simulink subsystem "Force_algebraic_estimator"  (R2021a)
settings: Solver=VariableStepAuto  StartTime=0.0  StopTime=10.0  RelTol=1e-3
values from neighbouring files (symbols this model uses):
  Af = 1.6    [kf_dict.sldd]
  Cd = 0.3    [kf_dict.sldd]
  rho_air = 1.206    [kf_dict.sldd]
undefined symbols (not defined in the file or in its folder): g, h, l, lf, lr, M, re
settings Model: Creator=Henrique Mesquita  LastModifiedBy=Henrique Mesquita

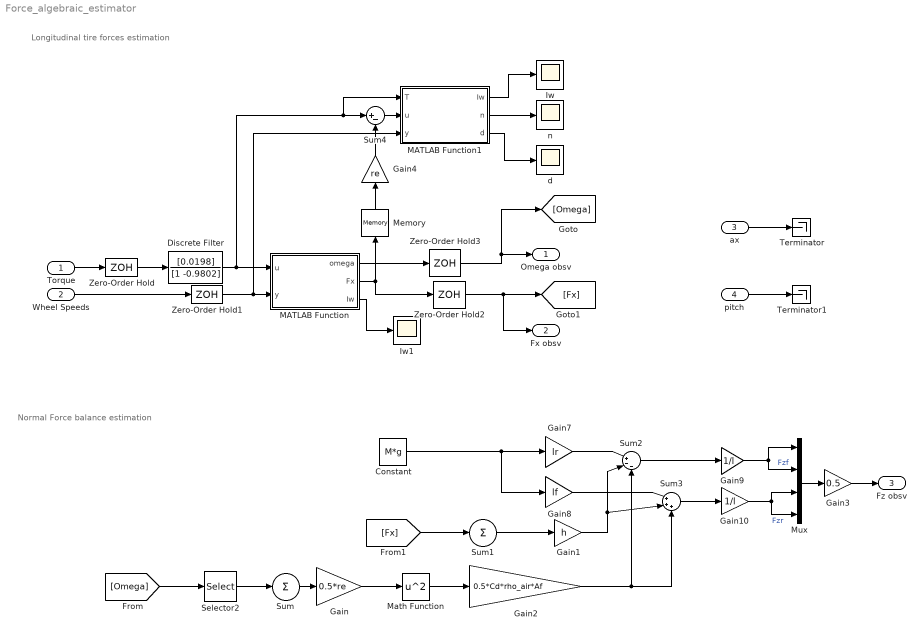
== system Force_algebraic_estimator ==
  note: Longitudinal tire forces estimation
  note: Normal Force balance estimation
  Torque : Inport  PortDimensions=4
  Wheel Speeds : Inport  Port=2  PortDimensions=4
  ax : Inport  Port=3  PortDimensions=1
  pitch : Inport  Port=4  PortDimensions=1
  Constant : Constant  Value=M*g
  Discrete Filter : DiscreteFilter  Numerator=[0.0198]  Denominator=[1 -0.9802]  SampleTime=0.001
  Gain : Gain  Gain=0.5*re
  Gain1 : Gain  Gain=h
  Gain10 : Gain  Gain=1/l
  Gain2 : Gain  Gain=0.5*Cd*rho_air*Af
  Gain3 : Gain  Gain=0.5
  Gain4 : Gain  Gain=re
  Gain7 : Gain  Gain=lr
  Gain8 : Gain  Gain=lf
  Gain9 : Gain  Gain=1/l
  Iw : Scope
  Iw1 : Scope
  MATLAB Function : MATLAB Function  TreatAsAtomicUnit=on
  MATLAB Function1 : MATLAB Function  TreatAsAtomicUnit=on
  Math Function : Math  Operator=square  SaturateOnIntegerOverflow=on
  Memory : Memory  LinearizeAsDelay=on
  Mux : Mux
  Selector2 : Selector  InputPortWidth=4  IndexOptions=Index vector (dialog)  Indices=[1 2]  OutputSizes=1
  Sum : Sum  Inputs=+
  Sum1 : Sum  Inputs=+
  Sum2 : Sum  Inputs=|+--
  Sum3 : Sum  Inputs=|+++
  Sum4 : Sum  Inputs=|+-
  Terminator : Terminator
  Terminator1 : Terminator
  Zero-Order Hold{,1..3} (4 alike) : ZeroOrderHold  SampleTime=0.001
  d : Scope
  n : Scope
  Omega obsv : Outport
  Fx obsv : Outport  Port=2
  Fz obsv : Outport  Port=3
  wires:
  Wheel Speeds/1 -> Zero-Order Hold1/1
  Zero-Order Hold2/1 -> [Fx], Fx obsv/1
  Zero-Order Hold3/1 -> Omega obsv/1, [Omega]
  ax/1 -> Terminator/1
  pitch/1 -> Terminator1/1
  [Omega] -> Selector2/1
  [Fx] -> Sum1/1
  Selector2/1 -> Sum/1
  Sum1/1 -> Gain1/1
  Sum/1 -> Gain/1
  Mux/1 -> Gain3/1
  Sum3/1 -> Gain10/1
  Gain10/1 -> Mux/3, Mux/4  "Fzr"
  Sum2/1 -> Gain9/1
  Gain1/1 -> Sum2/2, Sum3/2
  Gain9/1 -> Mux/1, Mux/2  "Fzf"
  Gain8/1 -> Sum3/1
  Gain7/1 -> Sum2/1
  Constant/1 -> Gain7/1, Gain8/1
  Gain/1 -> Math Function/1
  Math Function/1 -> Gain2/1
  Gain2/1 -> Sum2/3, Sum3/3
  Gain3/1 -> Fz obsv/1
  Torque/1 -> Zero-Order Hold/1
  Discrete Filter/1 -> MATLAB Function/1(u), Sum4/1, MATLAB Function1/1(T)
  Zero-Order Hold/1 -> Discrete Filter/1
  MATLAB Function/1(omega) -> Zero-Order Hold3/1
  Zero-Order Hold1/1 -> MATLAB Function/2(y), MATLAB Function1/3(y)
  MATLAB Function1/1(Iw) -> Iw/1
  MATLAB Function1/2(n) -> n/1
  MATLAB Function1/3(d) -> d/1
  Gain4/1 -> Sum4/2
  Memory/1 -> Gain4/1
  MATLAB Function/2(Fx) -> Memory/1, Zero-Order Hold2/1
  Sum4/1 -> MATLAB Function1/2(u)
  MATLAB Function/3(Iw) -> Iw1/1

== matlab function Force_algebraic_estimator/MATLAB Function ==
  settings: updateMethod=DISCRETE  sampleTime=0.001
  data: u input size=4; y input size=4; omega output size=4; Fx output size=4; Iw output size=4
function [omega, Fx, Iw] = fAlgEstimator(u, y)

N = 31;
Na = 151;
Ts = 0.001;
Ta = Na*Ts;
Jw = 0.8;
alpha = 1/Jw;
re = 0.284;
L = 1.25;

persistent y_mem;       % last output
persistent u_mem;       % last input
persistent phi_mem;
persistent omega_ant;
persistent phi_ant;
persistent alpha_ant;
persistent Nmax;
persistent s_y;
persistent s_u;
persistent s_ay;
persistent s_au;

if(isempty(y_mem)||isempty(u_mem))
    Nmax = max([N,Na]);
    y_mem = zeros(4,Nmax+1);
    u_mem = zeros(4,Nmax+1);
    phi_mem = zeros(4,Nmax+1);
    omega_ant = zeros(4,1);
    phi_ant = zeros(4,1);
    alpha_ant = 1/Jw*ones(4,1);
    
    %%% Early calculation and saving of the algebraic estimator coefficients
    T = N*Ts;
    i = N-1:-1:1;
    s_y = -6/T^3*[Ts/2*(T-2*N*Ts), Ts*(T-2*i*Ts), Ts/2*(T-2*0*Ts)];
    s_u = -6/T^3*[Ts/2*(T-N*Ts)*(N*Ts), Ts*(T-i*Ts).*(i*Ts), Ts/2*(T-0*Ts)*(0*Ts)];
    i = Na-1:-1:1;
    s_ay = [Ts/2*(0.5*Ta^2-2*Ta^2+1.5*Ta^2), Ts*(0.5*Ta^2-2*Ta*i*Ts+1.5*(i*Ts).^2), Ts/2*(0.5*Ta^2)];
    s_au = -[Ts/2*(Ta-Ta)^2*(Ta), Ts*((Ta-i*Ts).^2.*(i*Ts)), Ts/2*(Ta-0)^2*(0)];
    
%     s_ay = [Ts/2*(Ta^2-6*Ta*Na*Ts+6*(Na*Ts)^2), Ts*(Ta^2-6*Ta*i*Ts+6*(i*Ts).^2), Ts/2*(Ta^2-6*Ta*0*Ts+6*(0*Ts)^2)];
%     s_au = [Ts/2*(-Ta^2*Na*Ts+3*Ta*(Na*Ts)^2-2*(Na*Ts)^3), Ts*(-Ta^2*i*Ts+3*Ta*(i*Ts).^2-2*(i*Ts).^3), Ts/2*0];
end

%%% Wheel speed estimation
omega_bar = Ts*(phi_ant + alpha*u) +omega_ant;
omega = omega_bar + L*(y-omega_bar);
% omega = omega_bar;


for i = 0:Nmax-1
    u_mem(:,Nmax+1-i) = u_mem(:,Nmax-i);
    y_mem(:,Nmax+1-i) = y_mem(:,Nmax-i);
end
u_mem(:,1) = u;
y_mem(:,1) = y;

%%% Algebraic Estimation
phi=zeros(4,1);
du=zeros(4,1);
ny=zeros(4,1);
for i=1:Na+1
    du = du + s_au(i)*u_mem(:,i);
    ny = ny + s_ay(i)*y_mem(:,i);
end
for i=1:N+1
    phi = phi + (s_y(i)*y_mem(:,i) + alpha_ant.*s_u(i).*u_mem(:,i));
end
% phi= 6/T^3*(ny+du.*alpha_ant);
% phi = 6/T^3*phi;

% den = T^3/6*phi_ant-ny;
if(abs(du)<1e-2)
    alpha = alpha_ant;
else
    alpha = (Ta^4/24*phi_ant+ny)./du;
%     alpha = ny./du;
end
Iw=alpha;

Fx = -Jw/re*phi;

% alpha_ant = alpha;
omega_ant = omega;
phi_ant=phi;

== matlab function Force_algebraic_estimator/MATLAB Function1 ==
  settings: updateMethod=DISCRETE  sampleTime=0.001
  data: T input; u input size=4; y input size=4; Iw output size=4; n output size=4; d output size=4
function [Iw, n, d] = IwAlgEstimator(T, u, y)

Ts = 0.001;

persistent Iw0;
persistent t_ant;
persistent z_ant;
persistent eta_ant;
persistent y_ant;
persistent u_ant;

if(isempty(Iw0)||isempty(t_ant)||isempty(z_ant)||isempty(eta_ant)||isempty(y_ant)||isempty(u_ant))
    Iw0=0.8*ones(4,1);
    t_ant=0;
    z_ant = zeros(4,2);
    eta_ant = zeros(4,2);
    y_ant = zeros(4,1);
    u_ant = zeros(4,1);
    
end

t = t_ant + Ts;
z = zeros(4,2);
eta = zeros(4,2);

% z(:,2) = z_ant(:,2) + Ts/2*2*(y+y_ant);
% z(:,1) = z_ant(:,1) + Ts/2*(-4*(2*t-1)*(y+y_ant)+ (z(:,2) + z_ant(:,2)));
% n = t^2*y+z(:,1);
% 
% eta(:,2) = eta_ant(:,2) + Ts/2*(-2*t*u - 2*t_ant*u_ant);
% eta(:,1) = eta_ant(:,1) + Ts/2*(t^2*u + t_ant^2*u_ant+ (eta(:,2) + eta_ant(:,2)));
% d = eta(:,1);

%%% Backward euler integration
% z(:,2) = z_ant(:,2) + Ts*2*(y_ant);
% z(:,1) = z_ant(:,1) + Ts*(-4*t_ant*y_ant + z_ant(:,2));
% n = t^2*y+z(:,1);
% 
% eta(:,2) = eta_ant(:,2) + Ts*(2*t_ant*u_ant);
% eta(:,1) = eta_ant(:,1) + Ts*(t_ant^2*u_ant+ eta_ant(:,2));
% d = eta(:,1);

%%% Estimador sem integrador
% % z(:,2) = z_ant(:,2) + Ts/2*2*(y+y_ant);
% z(:,1) = z_ant(:,1) + Ts/2*(y+y_ant);
% n = -t*y+z(:,1);
% 
% % eta(:,2) = eta_ant(:,2) + Ts/2*(-2*t*u - 2*t_ant*u_ant);
% eta(:,1) = eta_ant(:,1) + Ts/2*(-t*u - t_ant*u_ant);
% d = eta(:,1);

%%% Estimador com integrador
z(:,2) = z_ant(:,2) + Ts/2*(y+y_ant);
z(:,1) = 0.1*z_ant(:,1) + Ts/2*(-t*y-t_ant*y_ant + z(:,2)+z_ant(:,2));
n = z(:,1);

eta(:,2) = eta_ant(:,2) + Ts/2*(-t*u - t_ant*u_ant);
eta(:,1) = 0.1*eta_ant(:,1) + Ts/2*(eta(:,2) + eta_ant(:,2));
d = eta(:,1);


if(t<0.2)
    Iw=Iw0;
elseif(abs(n)<1e-3)
    Iw=Iw0;
else
    Iw = d./n;
end

% if(t>3)
%     t=0;
%     Iw0=Iw;  
%     z = zeros(4,2);
%     eta = zeros(4,2);
% % elseif(T<10)
% %     t=0;
% %     Iw0=Iw;  
% %     z(3:4,:) = zeros(2,2);
% %     eta(3:4,:) = zeros(2,2);
% end

t_ant = t;
z_ant = z;
eta_ant = eta;
y_ant = y;
u_ant=u;
